simulink model "SingleTrack"  (R2019b)
settings: Solver=ode1  StartTime=0  StopTime=250  FixedStep=1.0000000000000000e-003  RelTol=1e-3
InitFcn:
  | sampleTime = str2double(get_param(bdroot, 'FixedStep'));
undefined symbols (not defined in the file or in its folder): AccPedalPos, BrakePedalPos, BrakeSwitch, DiscIntNeverNeededParam, DYNA4, EngSpd, IgnitionSwitch, InitialGear, InitialSpeed, IntendedEngTrq, LeftIndicator, MainBrakePress, MaxGear, MDL, MinGear, RefAcc, RefLane, RefLatPos, RefPath, RefPathCurv, RefSpd, RefSpdPreview, RefSpdRetrospect, RightIndicator, SteeringWheelAng, SteeringWheelTrq, UserDefinedRefValue, vm_const
libraries: UtilitiesLibrary x31, simulink x18, WheelSystemModules x13, LongitudinalControllerModules x13, LateralControllerModules x7, AnimationBusselectorModules x5, EnvironmentModules x5, BasicEngineControlModules x5, MiscellaneousControlModules x5, Animation3Modules x4, AuxiliariesModules x4, ReducedTireModules x4
(part 12 of 32)

== system SingleTrack/Vehicle/WheelSystem/FrontLeftWheelSystem ==
  note: These Signals are necessary for the Interaction with the Modular Drivetrain System.
  fromChassis : Inport
  fromCTRL : Inport  Port=2
  fromDrivetrain : Inport  Port=3
  fromBrakeSystem : Inport  Port=4
  BrakeTrqThresholdBlockingState : Constant  Value=0
  DynaSystemInfo : Subsystem  Tag=DynaSystemInfo
      mask init:
      | data = get_param(gcb, 'UserData');
      settings: OpenFcn=DYNA4.ModelHandling.System.ShowEditSystemInformationDialog(gcb);
      mask Display: disp(['Type = ', data.type, '\nName = ', data.name ])
  InnerTireOutput : Subsystem  Tag=TESIS DYNAware Interface Block  mask{NeedsUpdate=off, SignalInfo=|}
      mask SignalInfo=|
      | {
      |   "Version": "4.6",
      |   "MuxedOutputBusName": "Tire",
      |   "MuxedInputBusName": "input",
      |   "MuxedInputSelected": false,
      |   "MuxedOutputSelected": true,
      |   "SignalData": [
      |     {
      |       "initialValue": "0.0",
      |       "name": "",
      |       "comment": "",
      |       "minString": "",
      |       "maxString": "",
      |       "width": 3,
      |       "dataType": 0,
      |       "signalType": 0,
      |       "createSignal": true,
      |       "outputName": "ContactPointPos_wrt_WheelCenter(WorldSys)[m]",
      |       "generateSignalAccessBlock": false,
      |       "accessId": "$(parentId).$(blockName).$(outputName)"
      |     },
      |     {
      |       "initialValue": "0.0",
      |       "name": "",
      |       "comment": "",
      |       "minString": "",
      |       "maxString": "",
      |       "width": 1,
      |       "dataType": 0,
      |       "signalType": 0,
      |       "createSignal": true,
      |       "outputName": "CamberAng(ContactSys)[rad]",
      |       "generateSignalAccessBlock": false,
      |       "accessId": "$(parentId).$(blockName).$(outputName)"
      |     },
      |     {
      |       "initialValue": "0.0",
      |       "name": "",
      |       "comment": "",
      |       "minString": "",
      |       "maxString": "",
      |       "width": 1,
      |       "dataType": 0,
      |       "signalType": 0,
      |       "createSignal": true,
      |       "outputName": "TireDefl[m]",
      |       "generateSignalAccessBlock": false,
      |       "accessId": "$(parentId).$(blockName).$(outputName)"
      |     },
      |     {
      |       "initialValue": "0.0",
      |       "name": "",
      |       "comment": "",
      |       "minString": "",
      |       "maxString": "",
      |       "width": 1,
      |       "dataType": 0,
      |       "signalType": 0,
      |       "createSignal": true,
      |       "outputName": "TireDeflSpd[m/s]",
      |       "generateSignalAccessBlock": false,
      |       "accessId": "$(parentId).$(blockName).$(outputName)"
      |     },
      |     {
      |       "initialValue": "0.0",
      |       "name": "",
      |       "comment": "",
      |       "minString": "",
      |       "maxString": "",
      |       "width": 1,
      |       "dataType": 0,
      |       "signalType": 0,
      |       "createSignal": true,
      |       "outputName": "LongSpd(ContactSys)[m/s]",
      |       "generateSignalAccessBlock": false,
      |       "accessId": "$(parentId).$(blockName).$(outputName)"
      |     },
      |     {
      |       "initialValue": "0.0",
      |       "name": "",
      |       "comment": "",
      |       "minString": "",
      |       "maxString": "",
      |       "width": 1,
      |       "dataType": 0,
      |       "signalType": 0,
      |       "createSignal": true,
      |       "outputName": "LatSpd(ContactSys)[m/s]",
      |       "generateSignalAccessBlock": false,
      |       "accessId": "$(parentId).$(blockName).$(outputName)"
      |     },
      |     {
      |       "initialValue": "0.0",
      |       "name": "",
      |       "comment": "",
      |       "minString": "",
      |       "maxString": "",
      |       "width": 1,
      |       "dataType": 0,
      |       "signalType": 0,
      |       "createSignal": true,
      |       "outputName": "BoreSpd(ContactSys)[rad/s]",
      |       "generateSignalAccessBlock": false,
      |       "accessId": "$(parentId).$(blockName).$(outputName)"
      |     },
      |     {
      |       "initialValue": "0.0",
      |       "name": "",
      |       "comment": "",
      |       "minString": "",
      |       "maxString": "",
      |       "width": 1,
      |       "dataType": 0,
      |       "signalType": 0,
      |       "createSignal": true,
      |       "outputName": "LongFrcLeverArm_wrt_WheelRotAxis[m]",
      |       "generateSignalAccessBlock": false,
      |       "accessId": "$(parentId).$(blockName).$(outputName)"
      |     },
      |     {
      |       "initialValue": "0.0",
      |       "name": "",
      |       "comment": "",
      |       "minString": "",
      |       "maxString": "",
      |       "width": 3,
      |       "dataType": 0,
      |       "signalType": 0,
      |       "createSignal": true,
      |       "outputName": "LongUnitVector(WorldSys)[-]",
      |       "generateSignalAccessBlock": false,
      |       "accessId": "$(parentId).$(blockName).$(outputName)"
      |     },
      |     {
      |       "initialValue": "0.0",
      |       "name": "",
      |       "comment": "",
      |       "minString": "",
      |       "maxString": "",
      |       "width": 3,
      |       "dataType": 0,
      |       "signalType": 0,
      |       "createSignal": true,
      |       "outputName": "LatUnitVector(WorldSys)[-]",
      |       "generateSignalAccessBlock": false,
      |       "accessId": "$(parentId).$(blockName).$(outputName)"
      |     },
      |     {
      |       "initialValue": "0.0",
      |       "name": "",
      |       "comment": "",
      |       "minString": "",
      |       "maxString": "",
      |       "width": 3,
      |       "dataType": 0,
      |       "signalType": 0,
      |       "createSignal": true,
      |       "outputName": "RoadNormalVector(WorldSys)[-]",
      |       "generateSignalAccessBlock": false,
      |       "accessId": "$(parentId).$(blockName).$(outputName)"
      |     },
      |     {
      |       "initialValue": "0.0",
      |       "name": "",
      |       "comment": "",
      |       "minString": "",
      |       "maxString": "",
      |       "width": 1,
      |       "dataType": 0,
      |       "signalType": 0,
      |       "createSignal": true,
      |       "outputName": "RoadType[-]",
      |       "generateSignalAccessBlock": false,
      |       "accessId": "$(parentId).$(blockName).$(outputName)"
      |     },
      |     {
      |       "initialValue": "0.0",
      |       "name": "",
      |       "comment": "",
      |       "minString": "",
      |       "maxString": "",
      |       "width": 1,
      |       "dataType": 0,
      |       "signalType": 0,
      |       "createSignal": true,
      |       "outputName": "RoadFrictionScalingCoeff[-]",
      |       "generateSignalAccessBlock": false,
      |       "accessId": "$(parentId).$(blockName).$(outputName)"
      |     },
      |     {
      |       "initialValue": "0.0",
      |       "name": "",
      |       "comment": "",
      |       "minString": "",
      |       "maxString": "",
      |       "width": 3,
      |       "dataType": 0,
      |       "signalType": 0,
      |       "createSignal": true,
      |       "outputName": "ContactPointPos(WorldSys)[m]",
      |       "generateSignalAccessBlock": false,
      |       "accessId": "$(parentId).$(blockName).$(outputName)"
      |     },
      |     {
      |       "initialValue": "0.0",
      |       "name": "",
      |       "comment": "",
      |       "minString": "",
      |       "maxString": "",
      |       "width": 1,
      |       "dataType": 0,
      |       "signalType": 0,
      |       "createSignal": true,
      |       "outputName": "RoadSlope(WorldSys)[-]",
      |       "generateSignalAccessBlock": false,
      |       "accessId": "$(parentId).$(blockName).$(outputName)"
      |     },
      |     {
      |       "initialValue": "0.0",
      |       "name": "",
      |       "comment": "",
      |       "minString": "",
      |       "maxString": "",
      |       "width": 1,
      |       "dataType": 0,
      |       "signalType": 0,
      |       "createSignal": true,
      |       "outputName": "RoadIncl(WorldSys)[-]",
      |       "generateSignalAccessBlock": false,
      |       "accessId": "$(parentId).$(blockName).$(outputName)"
      |     },
      |     {
      |       "initialValue": "0.0",
      |       "name": "",
      |       "comment": "",
      |       "minString": "",
      |       "maxString": "",
      |       "width": 3,
      |       "dataType": 0,
      |       "signalType": 0,
      |       "createSignal": true,
      |       "outputName": "WheelCenterFrc(VehSys)[N]",
      |       "generateSignalAccessBlock": false,
      |       "accessId": "$(parentId).$(blockName).$(outputName)"
      |     },
      |     {
      |       "initialValue": "0.0",
      |       "name": "",
      |       "comment": "",
      |       "minString": "",
      |       "maxString": "",
      |       "width": 3,
      |       "dataType": 0,
      |       "signalType": 0,
      |       "createSignal": true,
      |       "outputName": "WheelCenterTrq(VehSys)[Nm]",
      |       "generateSignalAccessBlock": false,
      |       "accessId": "$(parentId).$(blockName).$(outputName)"
      |     },
      |     {
      |       "initialValue": "0.0",
      |       "name": "",
      |       "comment": "",
      |       "minString": "",
      |       "maxString": "",
      |       "width": 1,
      |       "dataType": 0,
      |       "signalType": 0,
      |       "createSignal": true,
      |       "outputName": "Stabilization.DerivativeOfLongFrc_wrt_LongSpd(ContactSys)[N/(m/s)]",
      |       "generateSignalAccessBlock": false,
      |       "accessId": "$(parentId).$(blockName).$(outputName)"
      |     },
      |     {
      |       "initialValue": "0.0",
      |       "name": "",
      |       "comment": "",
      |       "minString": "",
      |       "maxString": "",
      |       "width": 1,
      |       "dataType": 0,
      |       "signalType": 0,
      |       "createSignal": true,
      |       "outputName": "Stabilization.DerivativeOfLongTrq_wrt_LongSpd(ContactSys)[Nm/(m/s)]",
      |       "generateSignalAccessBlock": false,
      |       "accessId": "$(parentId).$(blockName).$(outputName)"
      |     },
      |     {
      |       "initialValue": "0.0",
      |       "name": "",
      |       "comment": "",
      |       "minString": "",
      |       "maxString": "",
      |       "width": 1,
      |       "dataType": 0,
      |       "signalType": 0,
      |       "createSignal": true,
      |       "outputName": "Stabilization.DerivativeOfLatFrc_wrt_LatSpd(ContactSys)[N/(m/s)]",
      |       "generateSignalAccessBlock": false,
      |       "accessId": "$(parentId).$(blockName).$(outputName)"
      |     },
      |     {
      |       "initialValue": "0.0",
      |       "name": "",
      |       "comment": "",
      |       "minString": "",
      |       "maxString": "",
      |       "width": 1,
      |       "dataType": 0,
      |       "signalType": 0,
      |       "createSignal": true,
      |       "outputName": "Stabilization.DerivativeOfLatTrq_wrt_LatSpd(ContactSys)[Nm/(m/s)]",
      |       "generateSignalAccessBlock": false,
      |       "accessId": "$(parentId).$(blockName).$(outputName)"
      |     },
      |     {
      |       "initialValue": "0.0",
      |       "name": "",
      |       "comment": "",
      |       "minString": "",
      |       "maxString": "",
      |       "width": 1,
      |       "dataType": 0,
      |       "signalType": 0,
      |       "createSignal": true,
      |       "outputName": "Stabilization.DerivativeOfBoreTrq_wrt_BoreSpd(ContactSys)[Nm/(rad/s)]",
      |       "generateSignalAccessBlock": false,
      |       "accessId": "$(parentId).$(blockName).$(outputName)"
      |     },
      |     {
      |       "initialValue": "0.0",
      |       "name": "",
      |       "comment": "",
      |       "minString": "",
      |       "maxString": "",
      |       "width": 1,
      |       "dataType": 0,
      |       "signalType": 0,
      |       "createSignal": true,
      |       "outputName": "CircumferentialTrq_wrt_WheelRotAxis[Nm]",
      |       "generateSignalAccessBlock": false,
      |       "accessId": "$(parentId).$(blockName).$(outputName)"
      |     },
      |     {
      |       "initialValue": "0.0",
      |       "name": "",
      |       "comment": "",
      |       "minString": "",
      |       "maxString": "",
      |       "width": 1,
      |       "dataType": 0,
      |       "signalType": 0,
      |       "createSignal": true,
      |       "outputName": "MaxRollResistTrq[Nm]",
      |       "generateSignalAccessBlock": false,
      |       "accessId": "$(parentId).$(blockName).$(outputName)"
      |     },
      |     {
      |       "initialValue": "0.0",
      |       "name": "",
      |       "comment": "",
      |       "minString": "",
      |       "maxString": "",
      |       "width": 1,
      |       "dataType": 0,
      |       "signalType": 0,
      |       "createSignal": true,
      |       "outputName": "LatDefl(ContactSys)[m]",
      |       "generateSignalAccessBlock": false,
      |       "accessId": "$(parentId).$(blockName).$(outputName)"
      |     },
      |     {
      |       "initialValue": "0.0",
      |       "name": "",
      |       "comment": "",
      |       "minString": "",
      |       "maxString": "",
      |       "width": 1,
      |       "dataType": 0,
      |       "signalType": 0,
      |       "createSignal": true,
      |       "outputName": "VertStiff[N/m]",
      |       "generateSignalAccessBlock": false,
      |       "accessId": "$(parentId).$(blockName).$(outputName)"
      |     },
      |     {
      |       "initialValue": "0.0",
      |       "name": "",
      |       "comment": "",
      |       "minString": "",
      |       "maxString": "",
      |       "width": 1,
      |       "dataType": 0,
      |       "signalType": 0,
      |       "createSignal": true,
      |       "outputName": "UnloadedRadius[m]",
      |       "generateSignalAccessBlock": false,
      |       "accessId": "$(parentId).$(blockName).$(outputName)"
      |     },
      |     {
      |       "initialValue": "0.0",
      |       "name": "",
      |       "comment": "",
      |       "minString": "",
      |       "maxString": "",
      |       "width": 1,
      |       "dataType": 0,
      |       "signalType": 0,
      |       "createSignal": true,
      |       "outputName": "RimRadius[m]",
      |       "generateSignalAccessBlock": false,
      |       "accessId": "$(parentId).$(blockName).$(outputName)"
      |     },
      |     {
      |       "initialValue": "0.0",
      |       "name": "",
      |       "comment": "",
      |       "minString": "",
      |       "maxString": "",
      |       "width": 1,
      |       "dataType": 0,
      |       "signalType": 0,
      |       "createSignal": true,
      |       "outputName": "Width[m]",
      |       "generateSignalAccessBlock": false,
      |       "accessId": "$(parentId).$(blockName).$(outputName)"
      |     },
      |     {
      |       "initialValue": "0.0",
      |       "name": "",
      |       "comment": "",
      |       "minString": "",
      |       "maxString": "",
      |       "width": 3,
      |       "dataType": 0,
      |       "signalType": 0,
      |       "createSignal": true,
      |       "outputName": "ContactPointFrc(ContactSys)[N]",
      |       "generateSignalAccessBlock": false,
      |       "accessId": "$(parentId).$(blockName).$(outputName)"
      |     },
      |     {
      |       "initialValue": "0.0",
      |       "name": "",
      |       "comment": "",
      |       "minString": "",
      |       "maxString": "",
      |       "width": 1,
      |       "dataType": 0,
      |       "signalType": 0,
      |       "createSignal": true,
      |       "outputName": "CorneringStiff[N]",
      |       "generateSignalAccessBlock": false,
      |       "accessId": "$(parentId).$(blockName).$(outputName)"
      |     },
      |     {
      |       "initialValue": "0.0",
      |       "name": "",
      |       "comment": "",
      |       "minString": "",
      |       "maxString": "",
      |       "width": 1,
      |       "dataType": 0,
      |       "signalType": 0,
      |       "createSignal": true,
      |       "outputName": "DynamicRadius[m]",
      |       "generateSignalAccessBlock": false,
      |       "accessId": "$(parentId).$(blockName).$(outputName)"
      |     }
      |   ]
      | }
      mask prompts: NeedsUpdate "Specify, if subsystem content needs to be updated"; SignalInfo "Signal Info (json)"
      mask help: DYNA4 Interface Block Version 4.6
      mask init:
      | blockName = get_param(gcbh, 'Name');
      | parentId = DYNA4.ModelHandling.AccessID.getFromHierarchy(gcbh);
      | TD.InterfaceBlock.ModelCallbacks.GenerateContent(gcb);
      settings: DeleteFcn=TD.InterfaceBlock.ModelCallbacks.CloseGUI( gcbh );  NameChangeFcn=TD.InterfaceBlock.ModelCallbacks.BlockRenamedHandler(gcbh);  OpenFcn=TD.InterfaceBlock.ModelCallbacks.OpenGUI( gcbh );  CloseFcn=TD.InterfaceBlock.ModelCallbacks.CloseGUI( gcbh );
      settings: AttributesFormatString=|
      | ContactPointPos_wrt_WheelCenter(WorldSys)[m] = 0.0
      | CamberAng(ContactSys)[rad] = 0.0
      | TireDefl[m] = 0.0
      | TireDeflSpd[m/s] = 0.0
      | ...
      mask Display:
      | image('InterfaceBlock.png','center');
      | port_label('output',1, 'Tire');
  KinematicWheelActiveFlag[0;1] : Constant  Value=0
  Tire : Subsystem
  TotalResistanceTorque : Constant  Value=0
  TraceMarker : UtilitiesLibrary/DYNA4 Trace Marker  Tag=DYNA4_TRACE_MARKER  SettingType=Custom  PrefixModelBlockID=on  PrefixRootSignalName=off  NamePattern='$(modelBlockID).Wheel'
  VehicleBodyReplacementInertia[kg*m**2] : Constant  Value=0
  Wheel : WheelSystemModules/Wheel  Tag=vedynaWheelMask  local_comp_inst=1  system_comp_inst=1  DATA_NODE=MDL.Vehicle.WheelSystem.FrontLeft.Wheel  sample_time=-1
  WheelInputs : WheelSystemModules/WheelInputs  SystemSampleTime=-1  Latency=0  AutoFrameSizeCalculation=off
  WheelOutput : Subsystem  Tag=TESIS DYNAware Interface Block  mask{NeedsUpdate=off, SignalInfo=|}
      mask SignalInfo=|
      | {
      |   "Version": "4.6",
      |   "MuxedOutputBusName": "Wheel",
      |   "MuxedInputBusName": "input",
      |   "MuxedInputSelected": false,
      |   "MuxedOutputSelected": true,
      |   "SignalData": [
      |     {
      |       "initialValue": "0.0",
      |       "name": "DriveBrakeTrq_wrt_WheelRotAxis(VehSys)[Nm]",
      |       "comment": "",
      |       "minString": "",
      |       "maxString": "",
      |       "width": 3,
      |       "dataType": 0,
      |       "signalType": 0,
      |       "createSignal": false,
      |       "outputName": "DriveBrakeTrq_wrt_WheelRotAxis(VehSys)[Nm]",
      |       "generateSignalAccessBlock": false,
      |       "accessId": "$(parentId).$(blockName).$(outputName)"
      |     },
      |     {
      |       "initialValue": "0.0",
      |       "name": "RotSpd[rad/s]",
      |       "comment": "",
      |       "minString": "",
      |       "maxString": "",
      |       "width": 1,
      |       "dataType": 0,
      |       "signalType": 0,
      |       "createSignal": false,
      |       "outputName": "RotSpd[rad/s]",
      |       "generateSignalAccessBlock": false,
      |       "accessId": "$(parentId).$(blockName).$(outputName)"
      |     },
      |     {
      |       "initialValue": "0.0",
      |       "name": "RotAcc[rad/s**2]",
      |       "comment": "",
      |       "minString": "",
      |       "maxString": "",
      |       "width": 1,
      |       "dataType": 0,
      |       "signalType": 0,
      |       "createSignal": false,
      |       "outputName": "RotAcc[rad/s**2]",
      |       "generateSignalAccessBlock": false,
      |       "accessId": "$(parentId).$(blockName).$(outputName)"
      |     },
      |     {
      |       "initialValue": "0.0",
      |       "name": "BlockingState[0;1]",
      |       "comment": "",
      |       "minString": "",
      |       "maxString": "",
      |       "width": 1,
      |       "dataType": 0,
      |       "signalType": 0,
      |       "createSignal": false,
      |       "outputName": "BlockingState[0;1]",
      |       "generateSignalAccessBlock": false,
      |       "accessId": "$(parentId).$(blockName).$(outputName)"
      |     },
      |     {
      |       "initialValue": "0.0",
      |       "name": "RotAng[rad]",
      |       "comment": "",
      |       "minString": "",
      |       "maxString": "",
      |       "width": 1,
      |       "dataType": 0,
      |       "signalType": 0,
      |       "createSignal": false,
      |       "outputName": "RotAng[rad]",
      |       "generateSignalAccessBlock": false,
      |       "accessId": "$(parentId).$(blockName).$(outputName)"
      |     },
      |     {
      |       "initialValue": "0.0",
      |       "name": "BrakeTrqPressRatio[m**3]",
      |       "comment": "",
      |       "minString": "",
      |       "maxString": "",
      |       "width": 1,
      |       "dataType": 0,
      |       "signalType": 0,
      |       "createSignal": false,
      |       "outputName": "BrakeTrqPressRatio[m**3]",
      |       "generateSignalAccessBlock": false,
      |       "accessId": "$(parentId).$(blockName).$(outputName)"
      |     },
      |     {
      |       "initialValue": "0.0",
      |       "name": "RotAxisInrt[kg*m**2]",
      |       "comment": "",
      |       "minString": "",
      |       "maxString": "",
      |       "width": 1,
      |       "dataType": 0,
      |       "signalType": 0,
      |       "createSignal": false,
      |       "outputName": "RotAxisInrt[kg*m**2]",
      |       "generateSignalAccessBlock": false,
      |       "accessId": "$(parentId).$(blockName).$(outputName)"
      |     },
      |     {
      |       "initialValue": "0.0",
      |       "name": "TotalResistanceTorque[Nm]",
      |       "comment": "",
      |       "minString": "",
      |       "maxString": "",
      |       "width": 1,
      |       "dataType": 0,
      |       "signalType": 0,
      |       "createSignal": false,
      |       "outputName": "TotalResistanceTorque[Nm]",
      |       "generateSignalAccessBlock": false,
      |       "accessId": "$(parentId).$(blockName).$(outputName)"
      |     },
      |     {
      |       "initialValue": "0.0",
      |       "name": "KinematicWheelActiveFlag[0;1]",
      |       "comment": "",
      |       "minString": "",
      |       "maxString": "",
      |       "width": 1,
      |       "dataType": 0,
      |       "signalType": 0,
      |       "createSignal": false,
      |       "outputName": "KinematicWheelActiveFlag[0;1]",
      |       "generateSignalAccessBlock": false,
      |       "accessId": "$(parentId).$(blockName).$(outputName)"
      |     },
      |     {
      |       "initialValue": "0.0",
      |       "name": "VehBodyReplacementInrt[kg*m**2]",
      |       "comment": "",
      |       "minString": "",
      |       "maxString": "",
      |       "width": 1,
      |       "dataType": 0,
      |       "signalType": 0,
      |       "createSignal": false,
      |       "outputName": "VehBodyReplacementInrt[kg*m**2]",
      |       "generateSignalAccessBlock": false,
      |       "accessId": "$(parentId).$(blockName).$(outputName)"
      |     }
      |   ]
      | }
      mask prompts: NeedsUpdate "Specify, if subsystem content needs to be updated"; SignalInfo "Signal Info (json)"
      mask help: DYNA4 Interface Block Version 4.6
      mask init:
      | blockName = get_param(gcbh, 'Name');
      | parentId = DYNA4.ModelHandling.AccessID.getFromHierarchy(gcbh);
      | TD.InterfaceBlock.ModelCallbacks.GenerateContent(gcb);
      settings: DeleteFcn=TD.InterfaceBlock.ModelCallbacks.CloseGUI( gcbh );  NameChangeFcn=TD.InterfaceBlock.ModelCallbacks.BlockRenamedHandler(gcbh);  OpenFcn=TD.InterfaceBlock.ModelCallbacks.OpenGUI( gcbh );  CloseFcn=TD.InterfaceBlock.ModelCallbacks.CloseGUI( gcbh );
      mask Display:
      | image('InterfaceBlock.png','center');
      | port_label('input',1, 'DriveBrakeTrq_wrt_WheelRotAxis(VehSys)[Nm]');
      | port_label('input',2, 'RotSpd[rad/s]');
      | port_label('input',3, 'RotAcc[rad/s**2]');
      | port_label('input',4, 'BlockingState[0;1]');
      | port_label('input',5, 'RotAng[rad]');
      | port_label('input',6, 'BrakeTrqPressRatio[m**3]');
      | port_label('input',7, 'RotAxisInrt[kg*m**2]');
      | port_label('input',8, 'TotalResistanceTorque[Nm]');
      | port_label('input',9, 'KinematicWheelActiveFlag[0;1]');
      | port_label('input',10, 'VehBodyReplacementInrt[kg*m**2]');
      | port_label('output',1, 'Wheel');
  InnerTireStates : Outport  VectorParamsAs1DForOutWhenUnconnected=off
  TireStates : Outport  Port=2  VectorParamsAs1DForOutWhenUnconnected=off
  WheelStates : Outport  Port=3  VectorParamsAs1DForOutWhenUnconnected=off
  wires:
  WheelInputs/1 -> Wheel/1
  WheelInputs/2 -> Wheel/2
  WheelInputs/3 -> Wheel/3
  WheelInputs/4 -> Wheel/4
  WheelInputs/5 -> Wheel/5
  WheelInputs/6 -> Wheel/6
  WheelInputs/7 -> Wheel/7
  WheelInputs/8 -> Wheel/8
  WheelInputs/9 -> Wheel/9
  WheelInputs/10 -> Wheel/10
  WheelInputs/11 -> Wheel/11
  WheelInputs/12 -> Wheel/12
  BrakeTrqThresholdBlockingState/1 -> Wheel/13
  VehicleBodyReplacementInertia[kg*m**2]/1 -> WheelOutput/10(VehBodyReplacementInrt[kg*m**2]___UNIQUE_1)
  KinematicWheelActiveFlag[0;1]/1 -> WheelOutput/9(KinematicWheelActiveFlag[0;1]___UNIQUE_1)
  TotalResistanceTorque/1 -> WheelOutput/8(TotalResistanceTorque[Nm]___UNIQUE_1)
  fromBrakeSystem/1 -> WheelInputs/6
  fromDrivetrain/1 -> WheelInputs/5
  fromCTRL/1 -> WheelInputs/3, Tire/1(fromCTRL)
  fromChassis/1 -> WheelInputs/4, Tire/2(fromChassis)
  InnerTireOutput/1(Tire___UNIQUE_1) -> WheelInputs/1, InnerTireStates/1
  Tire/1(Tire) -> WheelInputs/2, TireStates/1
  WheelOutput/1(Wheel___UNIQUE_1) -> Tire/3(fromWheel), WheelStates/1, TraceMarker/1
  Wheel/1 -> WheelOutput/1(DriveBrakeTrq_wrt_WheelRotAxis(VehSys)[Nm]___UNIQUE_1)
  Wheel/2 -> WheelOutput/2(RotSpd[rad/s]___UNIQUE_1)
  Wheel/3 -> WheelOutput/3(RotAcc[rad/s**2]___UNIQUE_1)
  Wheel/4 -> WheelOutput/4(BlockingState[0;1]___UNIQUE_1)
  Wheel/5 -> WheelOutput/5(RotAng[rad]___UNIQUE_1)
  Wheel/6 -> WheelOutput/6(BrakeTrqPressRatio[m**3]___UNIQUE_1)
  Wheel/7 -> WheelOutput/7(RotAxisInrt[kg*m**2]___UNIQUE_1)

== system SingleTrack/Vehicle/WheelSystem/FrontRightWheelSystem ==
  note: These Signals are necessary for the Interaction with the Modular Drivetrain System.
  fromChassis : Inport
  fromCTRL : Inport  Port=2
  fromDrivetrain : Inport  Port=3
  fromBrakeSystem : Inport  Port=4
  BrakeTrqThresholdBlockingState : Constant  Value=0
  DynaSystemInfo : Subsystem  Tag=DynaSystemInfo
      mask init:
      | data = get_param(gcb, 'UserData');
      settings: OpenFcn=DYNA4.ModelHandling.System.ShowEditSystemInformationDialog(gcb);
      mask Display: disp(['Type = ', data.type, '\nName = ', data.name ])
  InnerTireOutput : Subsystem  Tag=TESIS DYNAware Interface Block  mask{NeedsUpdate=off, SignalInfo=|}
      mask SignalInfo=|
      | {
      |   "Version": "4.6",
      |   "MuxedOutputBusName": "Tire",
      |   "MuxedInputBusName": "input",
      |   "MuxedInputSelected": false,
      |   "MuxedOutputSelected": true,
      |   "SignalData": [
      |     {
      |       "initialValue": "0.0",
      |       "name": "",
      |       "comment": "",
      |       "minString": "",
      |       "maxString": "",
      |       "width": 3,
      |       "dataType": 0,
      |       "signalType": 0,
      |       "createSignal": true,
      |       "outputName": "ContactPointPos_wrt_WheelCenter(WorldSys)[m]",
      |       "generateSignalAccessBlock": false,
      |       "accessId": "$(parentId).$(blockName).$(outputName)"
      |     },
      |     {
      |       "initialValue": "0.0",
      |       "name": "",
      |       "comment": "",
      |       "minString": "",
      |       "maxString": "",
      |       "width": 1,
      |       "dataType": 0,
      |       "signalType": 0,
      |       "createSignal": true,
      |       "outputName": "CamberAng(ContactSys)[rad]",
      |       "generateSignalAccessBlock": false,
      |       "accessId": "$(parentId).$(blockName).$(outputName)"
      |     },
      |     {
      |       "initialValue": "0.0",
      |       "name": "",
      |       "comment": "",
      |       "minString": "",
      |       "maxString": "",
      |       "width": 1,
      |       "dataType": 0,
      |       "signalType": 0,
      |       "createSignal": true,
      |       "outputName": "TireDefl[m]",
      |       "generateSignalAccessBlock": false,
      |       "accessId": "$(parentId).$(blockName).$(outputName)"
      |     },
      |     {
      |       "initialValue": "0.0",
      |       "name": "",
      |       "comment": "",
      |       "minString": "",
      |       "maxString": "",
      |       "width": 1,
      |       "dataType": 0,
      |       "signalType": 0,
      |       "createSignal": true,
      |       "outputName": "TireDeflSpd[m/s]",
      |       "generateSignalAccessBlock": false,
      |       "accessId": "$(parentId).$(blockName).$(outputName)"
      |     },
      |     {
      |       "initialValue": "0.0",
      |       "name": "",
      |       "comment": "",
      |       "minString": "",
      |       "maxString": "",
      |       "width": 1,
      |       "dataType": 0,
      |       "signalType": 0,
      |       "createSignal": true,
      |       "outputName": "LongSpd(ContactSys)[m/s]",
      |       "generateSignalAccessBlock": false,
      |       "accessId": "$(parentId).$(blockName).$(outputName)"
      |     },
      |     {
      |       "initialValue": "0.0",
      |       "name": "",
      |       "comment": "",
      |       "minString": "",
      |       "maxString": "",
      |       "width": 1,
      |       "dataType": 0,
      |       "signalType": 0,
      |       "createSignal": true,
      |       "outputName": "LatSpd(ContactSys)[m/s]",
      |       "generateSignalAccessBlock": false,
      |       "accessId": "$(parentId).$(blockName).$(outputName)"
      |     },
      |     {
      |       "initialValue": "0.0",
      |       "name": "",
      |       "comment": "",
      |       "minString": "",
      |       "maxString": "",
      |       "width": 1,
      |       "dataType": 0,
      |       "signalType": 0,
      |       "createSignal": true,
      |       "outputName": "BoreSpd(ContactSys)[rad/s]",
      |       "generateSignalAccessBlock": false,
      |       "accessId": "$(parentId).$(blockName).$(outputName)"
      |     },
      |     {
      |       "initialValue": "0.0",
      |       "name": "",
      |       "comment": "",
      |       "minString": "",
      |       "maxString": "",
      |       "width": 1,
      |       "dataType": 0,
      |       "signalType": 0,
      |       "createSignal": true,
      |       "outputName": "LongFrcLeverArm_wrt_WheelRotAxis[m]",
      |       "generateSignalAccessBlock": false,
      |       "accessId": "$(parentId).$(blockName).$(outputName)"
      |     },
      |     {
      |       "initialValue": "0.0",
      |       "name": "",
      |       "comment": "",
      |       "minString": "",
      |       "maxString": "",
      |       "width": 3,
      |       "dataType": 0,
      |       "signalType": 0,
      |       "createSignal": true,
      |       "outputName": "LongUnitVector(WorldSys)[-]",
      |       "generateSignalAccessBlock": false,
      |       "accessId": "$(parentId).$(blockName).$(outputName)"
      |     },
      |     {
      |       "initialValue": "0.0",
      |       "name": "",
      |       "comment": "",
      |       "minString": "",
      |       "maxString": "",
      |       "width": 3,
      |       "dataType": 0,
      |       "signalType": 0,
      |       "createSignal": true,
      |       "outputName": "LatUnitVector(WorldSys)[-]",
      |       "generateSignalAccessBlock": false,
      |       "accessId": "$(parentId).$(blockName).$(outputName)"
      |     },
      |     {
      |       "initialValue": "0.0",
      |       "name": "",
      |       "comment": "",
      |       "minString": "",
      |       "maxString": "",
      |       "width": 3,
      |       "dataType": 0,
      |       "signalType": 0,
      |       "createSignal": true,
      |       "outputName": "RoadNormalVector(WorldSys)[-]",
      |       "generateSignalAccessBlock": false,
      |       "accessId": "$(parentId).$(blockName).$(outputName)"
      |     },
      |     {
      |       "initialValue": "0.0",
      |       "name": "",
      |       "comment": "",
      |       "minString": "",
      |       "maxString": "",
      |       "width": 1,
      |       "dataType": 0,
      |       "signalType": 0,
      |       "createSignal": true,
      |       "outputName": "RoadType[-]",
      |       "generateSignalAccessBlock": false,
      |       "accessId": "$(parentId).$(blockName).$(outputName)"
      |     },
      |     {
      |       "initialValue": "0.0",
      |       "name": "",
      |       "comment": "",
      |       "minString": "",
      |       "maxString": "",
      |       "width": 1,
      |       "dataType": 0,
      |       "signalType": 0,
      |       "createSignal": true,
      |       "outputName": "RoadFrictionScalingCoeff[-]",
      |       "generateSignalAccessBlock": false,
      |       "accessId": "$(parentId).$(blockName).$(outputName)"
      |     },
      |     {
      |       "initialValue": "0.0",
      |       "name": "",
      |       "comment": "",
      |       "minString": "",
      |       "maxString": "",
      |       "width": 3,
      |       "dataType": 0,
      |       "signalType": 0,
      |       "createSignal": true,
      |       "outputName": "ContactPointPos(WorldSys)[m]",
      |       "generateSignalAccessBlock": false,
      |       "accessId": "$(parentId).$(blockName).$(outputName)"
      |     },
      |     {
      |       "initialValue": "0.0",
      |       "name": "",
      |       "comment": "",
      |       "minString": "",
      |       "maxString": "",
      |       "width": 1,
      |       "dataType": 0,
      |       "signalType": 0,
      |       "createSignal": true,
      |       "outputName": "RoadSlope(WorldSys)[-]",
      |       "generateSignalAccessBlock": false,
      |       "accessId": "$(parentId).$(blockName).$(outputName)"
      |     },
      |     {
      |       "initialValue": "0.0",
      |       "name": "",
      |       "comment": "",
      |       "minString": "",
      |       "maxString": "",
      |       "width": 1,
      |       "dataType": 0,
      |       "signalType": 0,
      |       "createSignal": true,
      |       "outputName": "RoadIncl(WorldSys)[-]",
      |       "generateSignalAccessBlock": false,
      |       "accessId": "$(parentId).$(blockName).$(outputName)"
      |     },
      |     {
      |       "initialValue": "0.0",
      |       "name": "",
      |       "comment": "",
      |       "minString": "",
      |       "maxString": "",
      |       "width": 3,
      |       "dataType": 0,
      |       "signalType": 0,
      |       "createSignal": true,
      |       "outputName": "WheelCenterFrc(VehSys)[N]",
      |       "generateSignalAccessBlock": false,
      |       "accessId": "$(parentId).$(blockName).$(outputName)"
      |     },
      |     {
      |       "initialValue": "0.0",
      |       "name": "",
      |       "comment": "",
      |       "minString": "",
      |       "maxString": "",
      |       "width": 3,
      |       "dataType": 0,
      |       "signalType": 0,
      |       "createSignal": true,
      |       "outputName": "WheelCenterTrq(VehSys)[Nm]",
      |       "generateSignalAccessBlock": false,
      |       "accessId": "$(parentId).$(blockName).$(outputName)"
      |     },
      |     {
      |       "initialValue": "0.0",
      |       "name": "",
      |       "comment": "",
      |       "minString": "",
      |       "maxString": "",
      |       "width": 1,
      |       "dataType": 0,
      |       "signalType": 0,
      |       "createSignal": true,
      |       "outputName": "Stabilization.DerivativeOfLongFrc_wrt_LongSpd(ContactSys)[N/(m/s)]",
      |       "generateSignalAccessBlock": false,
      |       "accessId": "$(parentId).$(blockName).$(outputName)"
      |     },
      |     {
      |       "initialValue": "0.0",
      |       "name": "",
      |       "comment": "",
      |       "minString": "",
      |       "maxString": "",
      |       "width": 1,
      |       "dataType": 0,
      |       "signalType": 0,
      |       "createSignal": true,
      |       "outputName": "Stabilization.DerivativeOfLongTrq_wrt_LongSpd(ContactSys)[Nm/(m/s)]",
      |       "generateSignalAccessBlock": false,
      |       "accessId": "$(parentId).$(blockName).$(outputName)"
      |     },
      |     {
      |       "initialValue": "0.0",
      |       "name": "",
      |       "comment": "",
      |       "minString": "",
      |       "maxString": "",
      |       "width": 1,
      |       "dataType": 0,
      |       "signalType": 0,
      |       "createSignal": true,
      |       "outputName": "Stabilization.DerivativeOfLatFrc_wrt_LatSpd(ContactSys)[N/(m/s)]",
      |       "generateSignalAccessBlock": false,
      |       "accessId": "$(parentId).$(blockName).$(outputName)"
      |     },
      |     {
      |       "initialValue": "0.0",
      |       "name": "",
      |       "comment": "",
      |       "minString": "",
      |       "maxString": "",
      |       "width": 1,
      |       "dataType": 0,
      |       "signalType": 0,
      |       "createSignal": true,
      |       "outputName": "Stabilization.DerivativeOfLatTrq_wrt_LatSpd(ContactSys)[Nm/(m/s)]",
      |       "generateSignalAccessBlock": false,
      |       "accessId": "$(parentId).$(blockName).$(outputName)"
      |     },
      |     {
      |       "initialValue": "0.0",
      |       "name": "",
      |       "comment": "",
      |       "minString": "",
      |       "maxString": "",
      |       "width": 1,
      |       "dataType": 0,
      |       "signalType": 0,
      |       "createSignal": true,
      |       "outputName": "Stabilization.DerivativeOfBoreTrq_wrt_BoreSpd(ContactSys)[Nm/(rad/s)]",
      |       "generateSignalAccessBlock": false,
      |       "accessId": "$(parentId).$(blockName).$(outputName)"
      |     },
      |     {
      |       "initialValue": "0.0",
      |       "name": "",
      |       "comment": "",
      |       "minString": "",
      |       "maxString": "",
      |       "width": 1,
      |       "dataType": 0,
      |       "signalType": 0,
      |       "createSignal": true,
      |       "outputName": "CircumferentialTrq_wrt_WheelRotAxis[Nm]",
      |       "generateSignalAccessBlock": false,
      |       "accessId": "$(parentId).$(blockName).$(outputName)"
      |     },
      |     {
      |       "initialValue": "0.0",
      |       "name": "",
      |       "comment": "",
      |       "minString": "",
      |       "maxString": "",
      |       "width": 1,
      |       "dataType": 0,
      |       "signalType": 0,
      |       "createSignal": true,
      |       "outputName": "MaxRollResistTrq[Nm]",
      |       "generateSignalAccessBlock": false,
      |       "accessId": "$(parentId).$(blockName).$(outputName)"
      |     },
      |     {
      |       "initialValue": "0.0",
      |       "name": "",
      |       "comment": "",
      |       "minString": "",
      |       "maxString": "",
      |       "width": 1,
      |       "dataType": 0,
      |       "signalType": 0,
      |       "createSignal": true,
      |       "outputName": "LatDefl(ContactSys)[m]",
      |       "generateSignalAccessBlock": false,
      |       "accessId": "$(parentId).$(blockName).$(outputName)"
      |     },
      |     {
      |       "initialValue": "0.0",
      |       "name": "",
      |       "comment": "",
      |       "minString": "",
      |       "maxString": "",
      |       "width": 1,
      |       "dataType": 0,
      |       "signalType": 0,
      |       "createSignal": true,
      |       "outputName": "VertStiff[N/m]",
      |       "generateSignalAccessBlock": false,
      |       "accessId": "$(parentId).$(blockName).$(outputName)"
      |     },
      |     {
      |       "initialValue": "0.0",
      |       "name": "",
      |       "comment": "",
      |       "minString": "",
      |       "maxString": "",
      |       "width": 1,
      |       "dataType": 0,
      |       "signalType": 0,
      |       "createSignal": true,
      |       "outputName": "UnloadedRadius[m]",
      |       "generateSignalAccessBlock": false,
      |       "accessId": "$(parentId).$(blockName).$(outputName)"
      |     },
      |     {
      |       "initialValue": "0.0",
      |       "name": "",
      |       "comment": "",
      |       "minString": "",
      |       "maxString": "",
      |       "width": 1,
      |       "dataType": 0,
      |       "signalType": 0,
      |       "createSignal": true,
      |       "outputName": "RimRadius[m]",
      |       "generateSignalAccessBlock": false,
      |       "accessId": "$(parentId).$(blockName).$(outputName)"
      |     },
      |     {
      |       "initialValue": "0.0",
      |       "name": "",
      |       "comment": "",
      |       "minString": "",
      |       "maxString": "",
      |       "width": 1,
      |       "dataType": 0,
      |       "signalType": 0,
      |       "createSignal": true,
      |       "outputName": "Width[m]",
      |       "generateSignalAccessBlock": false,
      |       "accessId": "$(parentId).$(blockName).$(outputName)"
      |     },
      |     {
      |       "initialValue": "0.0",
      |       "name": "",
      |       "comment": "",
      |       "minString": "",
      |       "maxString": "",
      |       "width": 3,
      |       "dataType": 0,
      |       "signalType": 0,
      |       "createSignal": true,
      |       "outputName": "ContactPointFrc(ContactSys)[N]",
      |       "generateSignalAccessBlock": false,
      |       "accessId": "$(parentId).$(blockName).$(outputName)"
      |     },
      |     {
      |       "initialValue": "0.0",
      |       "name": "",
      |       "comment": "",
      |       "minString": "",
      |       "maxString": "",
      |       "width": 1,
      |       "dataType": 0,
      |       "signalType": 0,
      |       "createSignal": true,
      |       "outputName": "CorneringStiff[N]",
      |       "generateSignalAccessBlock": false,
      |       "accessId": "$(parentId).$(blockName).$(outputName)"
      |     },
      |     {
      |       "initialValue": "0.0",
      |       "name": "",
      |       "comment": "",
      |       "minString": "",
      |       "maxString": "",
      |       "width": 1,
      |       "dataType": 0,
      |       "signalType": 0,
      |       "createSignal": true,
      |       "outputName": "DynamicRadius[m]",
      |       "generateSignalAccessBlock": false,
      |       "accessId": "$(parentId).$(blockName).$(outputName)"
      |     }
      |   ]
      | }
      mask prompts: NeedsUpdate "Specify, if subsystem content needs to be updated"; SignalInfo "Signal Info (json)"
      mask help: DYNA4 Interface Block Version 4.6
      mask init:
      | blockName = get_param(gcbh, 'Name');
      | parentId = DYNA4.ModelHandling.AccessID.getFromHierarchy(gcbh);
      | TD.InterfaceBlock.ModelCallbacks.GenerateContent(gcb);
      settings: DeleteFcn=TD.InterfaceBlock.ModelCallbacks.CloseGUI( gcbh );  NameChangeFcn=TD.InterfaceBlock.ModelCallbacks.BlockRenamedHandler(gcbh);  OpenFcn=TD.InterfaceBlock.ModelCallbacks.OpenGUI( gcbh );  CloseFcn=TD.InterfaceBlock.ModelCallbacks.CloseGUI( gcbh );
      settings: AttributesFormatString=|
      | ContactPointPos_wrt_WheelCenter(WorldSys)[m] = 0.0
      | CamberAng(ContactSys)[rad] = 0.0
      | TireDefl[m] = 0.0
      | TireDeflSpd[m/s] = 0.0
      | ...
      mask Display:
      | image('InterfaceBlock.png','center');
      | port_label('output',1, 'Tire');
  KinematicWheelActiveFlag[0;1] : Constant  Value=0
  Tire : Subsystem
  TotalResistanceTorque : Constant  Value=0
  TraceMarker : UtilitiesLibrary/DYNA4 Trace Marker  Tag=DYNA4_TRACE_MARKER  SettingType=Custom  PrefixModelBlockID=on  PrefixRootSignalName=off  NamePattern='$(modelBlockID).Wheel'
  VehicleBodyReplacementInertia[kg*m**2] : Constant  Value=0
  Wheel : WheelSystemModules/Wheel  Tag=vedynaWheelMask  local_comp_inst=2  system_comp_inst=2  DATA_NODE=MDL.Vehicle.WheelSystem.FrontRight.Wheel  sample_time=-1
  WheelInputs : WheelSystemModules/WheelInputs  SystemSampleTime=-1  Latency=0  AutoFrameSizeCalculation=off
  WheelOutput : Subsystem  Tag=TESIS DYNAware Interface Block  mask{NeedsUpdate=off, SignalInfo=|}
      mask SignalInfo=|
      | {
      |   "Version": "4.6",
      |   "MuxedOutputBusName": "Wheel",
      |   "MuxedInputBusName": "input",
      |   "MuxedInputSelected": false,
      |   "MuxedOutputSelected": true,
      |   "SignalData": [
      |     {
      |       "initialValue": "0.0",
      |       "name": "DriveBrakeTrq_wrt_WheelRotAxis(VehSys)[Nm]",
      |       "comment": "",
      |       "minString": "",
      |       "maxString": "",
      |       "width": 3,
      |       "dataType": 0,
      |       "signalType": 0,
      |       "createSignal": false,
      |       "outputName": "DriveBrakeTrq_wrt_WheelRotAxis(VehSys)[Nm]",
      |       "generateSignalAccessBlock": false,
      |       "accessId": "$(parentId).$(blockName).$(outputName)"
      |     },
      |     {
      |       "initialValue": "0.0",
      |       "name": "RotSpd[rad/s]",
      |       "comment": "",
      |       "minString": "",
      |       "maxString": "",
      |       "width": 1,
      |       "dataType": 0,
      |       "signalType": 0,
      |       "createSignal": false,
      |       "outputName": "RotSpd[rad/s]",
      |       "generateSignalAccessBlock": false,
      |       "accessId": "$(parentId).$(blockName).$(outputName)"
      |     },
      |     {
      |       "initialValue": "0.0",
      |       "name": "RotAcc[rad/s**2]",
      |       "comment": "",
      |       "minString": "",
      |       "maxString": "",
      |       "width": 1,
      |       "dataType": 0,
      |       "signalType": 0,
      |       "createSignal": false,
      |       "outputName": "RotAcc[rad/s**2]",
      |       "generateSignalAccessBlock": false,
      |       "accessId": "$(parentId).$(blockName).$(outputName)"
      |     },
      |     {
      |       "initialValue": "0.0",
      |       "name": "BlockingState[0;1]",
      |       "comment": "",
      |       "minString": "",
      |       "maxString": "",
      |       "width": 1,
      |       "dataType": 0,
      |       "signalType": 0,
      |       "createSignal": false,
      |       "outputName": "BlockingState[0;1]",
      |       "generateSignalAccessBlock": false,
      |       "accessId": "$(parentId).$(blockName).$(outputName)"
      |     },
      |     {
      |       "initialValue": "0.0",
      |       "name": "RotAng[rad]",
      |       "comment": "",
      |       "minString": "",
      |       "maxString": "",
      |       "width": 1,
      |       "dataType": 0,
      |       "signalType": 0,
      |       "createSignal": false,
      |       "outputName": "RotAng[rad]",
      |       "generateSignalAccessBlock": false,
      |       "accessId": "$(parentId).$(blockName).$(outputName)"
      |     },
      |     {
      |       "initialValue": "0.0",
      |       "name": "BrakeTrqPressRatio[m**3]",
      |       "comment": "",
      |       "minString": "",
      |       "maxString": "",
      |       "width": 1,
      |       "dataType": 0,
      |       "signalType": 0,
      |       "createSignal": false,
      |       "outputName": "BrakeTrqPressRatio[m**3]",
      |       "generateSignalAccessBlock": false,
      |       "accessId": "$(parentId).$(blockName).$(outputName)"
      |     },
      |     {
      |       "initialValue": "0.0",
      |       "name": "RotAxisInrt[kg*m**2]",
      |       "comment": "",
      |       "minString": "",
      |       "maxString": "",
      |       "width": 1,
      |       "dataType": 0,
      |       "signalType": 0,
      |       "createSignal": false,
      |       "outputName": "RotAxisInrt[kg*m**2]",
      |       "generateSignalAccessBlock": false,
      |       "accessId": "$(parentId).$(blockName).$(outputName)"
      |     },
      |     {
      |       "initialValue": "0.0",
      |       "name": "TotalResistanceTorque[Nm]",
      |       "comment": "",
      |       "minString": "",
      |       "maxString": "",
      |       "width": 1,
      |       "dataType": 0,
      |       "signalType": 0,
      |       "createSignal": false,
      |       "outputName": "TotalResistanceTorque[Nm]",
      |       "generateSignalAccessBlock": false,
      |       "accessId": "$(parentId).$(blockName).$(outputName)"
      |     },
      |     {
      |       "initialValue": "0.0",
      |       "name": "KinematicWheelActiveFlag[0;1]",
      |       "comment": "",
      |       "minString": "",
      |       "maxString": "",
      |       "width": 1,
      |       "dataType": 0,
      |       "signalType": 0,
      |       "createSignal": false,
      |       "outputName": "KinematicWheelActiveFlag[0;1]",
      |       "generateSignalAccessBlock": false,
      |       "accessId": "$(parentId).$(blockName).$(outputName)"
      |     },
      |     {
      |       "initialValue": "0.0",
      |       "name": "VehBodyReplacementInrt[kg*m**2]",
      |       "comment": "",
      |       "minString": "",
      |       "maxString": "",
      |       "width": 1,
      |       "dataType": 0,
      |       "signalType": 0,
      |       "createSignal": false,
      |       "outputName": "VehBodyReplacementInrt[kg*m**2]",
      |       "generateSignalAccessBlock": false,
      |       "accessId": "$(parentId).$(blockName).$(outputName)"
      |     }
      |   ]
      | }
      mask prompts: NeedsUpdate "Specify, if subsystem content needs to be updated"; SignalInfo "Signal Info (json)"
      mask help: DYNA4 Interface Block Version 4.6
      mask init:
      | blockName = get_param(gcbh, 'Name');
      | parentId = DYNA4.ModelHandling.AccessID.getFromHierarchy(gcbh);
      | TD.InterfaceBlock.ModelCallbacks.GenerateContent(gcb);
      settings: DeleteFcn=TD.InterfaceBlock.ModelCallbacks.CloseGUI( gcbh );  NameChangeFcn=TD.InterfaceBlock.ModelCallbacks.BlockRenamedHandler(gcbh);  OpenFcn=TD.InterfaceBlock.ModelCallbacks.OpenGUI( gcbh );  CloseFcn=TD.InterfaceBlock.ModelCallbacks.CloseGUI( gcbh );
      mask Display:
      | image('InterfaceBlock.png','center');
      | port_label('input',1, 'DriveBrakeTrq_wrt_WheelRotAxis(VehSys)[Nm]');
      | port_label('input',2, 'RotSpd[rad/s]');
      | port_label('input',3, 'RotAcc[rad/s**2]');
      | port_label('input',4, 'BlockingState[0;1]');
      | port_label('input',5, 'RotAng[rad]');
      | port_label('input',6, 'BrakeTrqPressRatio[m**3]');
      | port_label('input',7, 'RotAxisInrt[kg*m**2]');
      | port_label('input',8, 'TotalResistanceTorque[Nm]');
      | port_label('input',9, 'KinematicWheelActiveFlag[0;1]');
      | port_label('input',10, 'VehBodyReplacementInrt[kg*m**2]');
      | port_label('output',1, 'Wheel');
  InnerTireStates : Outport  VectorParamsAs1DForOutWhenUnconnected=off
  TireStates : Outport  Port=2  VectorParamsAs1DForOutWhenUnconnected=off
  WheelStates : Outport  Port=3  VectorParamsAs1DForOutWhenUnconnected=off
  wires:
  BrakeTrqThresholdBlockingState/1 -> Wheel/13
  WheelInputs/12 -> Wheel/12
  WheelInputs/11 -> Wheel/11
  WheelInputs/10 -> Wheel/10
  WheelInputs/9 -> Wheel/9
  WheelInputs/8 -> Wheel/8
  WheelInputs/7 -> Wheel/7
  WheelInputs/6 -> Wheel/6
  WheelInputs/5 -> Wheel/5
  WheelInputs/4 -> Wheel/4
  WheelInputs/3 -> Wheel/3
  WheelInputs/2 -> Wheel/2
  WheelInputs/1 -> Wheel/1
  VehicleBodyReplacementInertia[kg*m**2]/1 -> WheelOutput/10(VehBodyReplacementInrt[kg*m**2]___UNIQUE_1)
  KinematicWheelActiveFlag[0;1]/1 -> WheelOutput/9(KinematicWheelActiveFlag[0;1]___UNIQUE_1)
  TotalResistanceTorque/1 -> WheelOutput/8(TotalResistanceTorque[Nm]___UNIQUE_1)
  Wheel/7 -> WheelOutput/7(RotAxisInrt[kg*m**2]___UNIQUE_1)
  Wheel/6 -> WheelOutput/6(BrakeTrqPressRatio[m**3]___UNIQUE_1)
  Wheel/5 -> WheelOutput/5(RotAng[rad]___UNIQUE_1)
  Wheel/4 -> WheelOutput/4(BlockingState[0;1]___UNIQUE_1)
  Wheel/3 -> WheelOutput/3(RotAcc[rad/s**2]___UNIQUE_1)
  Wheel/2 -> WheelOutput/2(RotSpd[rad/s]___UNIQUE_1)
  Wheel/1 -> WheelOutput/1(DriveBrakeTrq_wrt_WheelRotAxis(VehSys)[Nm]___UNIQUE_1)
  WheelOutput/1(Wheel___UNIQUE_1) -> Tire/3(fromWheel), WheelStates/1, TraceMarker/1
  Tire/1(Tire) -> WheelInputs/2, TireStates/1
  InnerTireOutput/1(Tire___UNIQUE_1) -> WheelInputs/1, InnerTireStates/1
  fromChassis/1 -> Tire/2(fromChassis), WheelInputs/4
  fromCTRL/1 -> Tire/1(fromCTRL), WheelInputs/3
  fromDrivetrain/1 -> WheelInputs/5
  fromBrakeSystem/1 -> WheelInputs/6
